simulink model "motivation"  (R2021b)
settings: Solver=FixedStepAuto  StartTime=0.0  StopTime=simTime  FixedStep=simStep  RelTol=1e-3
values from neighbouring files (symbols this model uses):
  Delta = 0.1    [init.m]
  Gain = place(A,b, [-3 , -10])    [init.m]
  Gains = place(As, bs, [0.2 , 0.1])    [init.m]
  k1 = 1    [init.m]
  k2 = 1    [init.m]
  simStep = 10^-4    (= 0.0001)    [init.m]
  x0 = [-1;1]    [init.m]
settings Model: Creator=mebbaid  LastModifiedBy=mebbaid

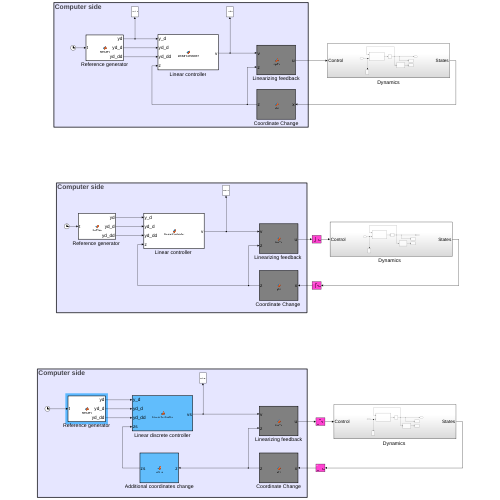
[thumbnail: Simulink's stored preview of the top-level diagram]
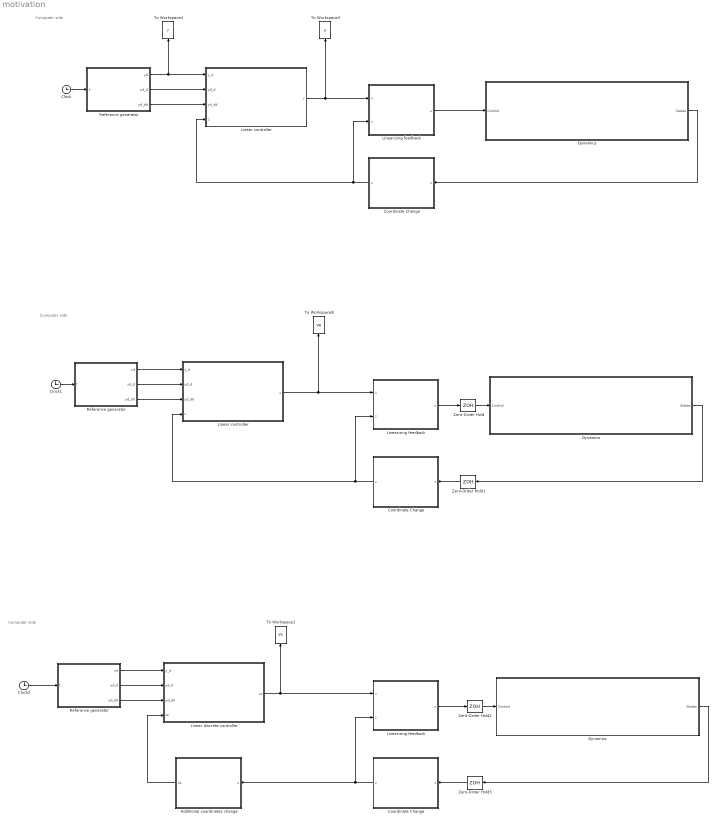
== system motivation ==
  note: Computer side
  note: Computer side
  note: Computer side
  " Coordinate Change " : MATLAB Function  TreatAsAtomicUnit=on
  " Dynamics  " : Subsystem
  " Linearizing feedback " : MATLAB Function  TreatAsAtomicUnit=on
  " Reference generator " : MATLAB Function  TreatAsAtomicUnit=on
  Additional coordinates change : MATLAB Function  TreatAsAtomicUnit=on
  Clock : Clock
  Clock1 : Clock
  Clock2 : Clock
  Coordinate Change : MATLAB Function  TreatAsAtomicUnit=on
  "Coordinate Change " : MATLAB Function  TreatAsAtomicUnit=on
  Dynamics : Subsystem
  "Dynamics  " : Subsystem
  Linear controller : MATLAB Function  TreatAsAtomicUnit=on
  "Linear controller " : MATLAB Function  TreatAsAtomicUnit=on
  Linear discrete controller : MATLAB Function  TreatAsAtomicUnit=on
  Linearizing feedback : MATLAB Function  TreatAsAtomicUnit=on
  "Linearizing feedback " : MATLAB Function  TreatAsAtomicUnit=on
  Reference generator : MATLAB Function  TreatAsAtomicUnit=on
  "Reference generator " : MATLAB Function  TreatAsAtomicUnit=on
  To Workspace1 : ToWorkspace  VariableName=vs  SaveFormat=Timeseries  SampleTime=simStep
      settings: Save2DSignal=2-D array (concatenate along first dimension)
  To Workspace3 : ToWorkspace  VariableName=v  SaveFormat=Timeseries  SampleTime=simStep
      settings: Save2DSignal=2-D array (concatenate along first dimension)
  To Workspace4 : ToWorkspace  VariableName=r  SaveFormat=Timeseries  SampleTime=simStep
      settings: Save2DSignal=2-D array (concatenate along first dimension)
  To Workspace8 : ToWorkspace  VariableName=ve  SaveFormat=Timeseries  SampleTime=simStep
      settings: Save2DSignal=2-D array (concatenate along first dimension)
  Zero-Order Hold{,1..3} (4 alike) : ZeroOrderHold  SampleTime=Delta
  wires:
  Linear controller/1(v) -> Linearizing feedback/1(v), To Workspace3/1
  Clock/1 -> Reference generator/1(t)
  Reference generator/3(yd_dd) -> Linear controller/3(yd_dd)
  Reference generator/1(yd) -> Linear controller/1(y_d), To Workspace4/1
  Reference generator/2(yd_d) -> Linear controller/2(yd_d)
  Linearizing feedback/1(u) -> Dynamics/1(Control)
  Coordinate Change/1(z) -> Linear controller/4(z), Linearizing feedback/2(z)
  Dynamics/1(States) -> Coordinate Change/1(x)
  "Linearizing feedback "/1(u) -> Zero-Order Hold/1
  "Dynamics  "/1(States) -> Zero-Order Hold1/1
  "Linear controller "/1(v) -> "Linearizing feedback "/1(v), To Workspace8/1
  "Coordinate Change "/1(z) -> "Linear controller "/4(z), "Linearizing feedback "/2(z)
  "Reference generator "/1(yd) -> "Linear controller "/1(y_d)
  "Reference generator "/2(yd_d) -> "Linear controller "/2(yd_d)
  "Reference generator "/3(yd_dd) -> "Linear controller "/3(yd_dd)
  Clock1/1 -> "Reference generator "/1(t)
  Zero-Order Hold/1 -> "Dynamics  "/1(Control)
  Zero-Order Hold1/1 -> "Coordinate Change "/1(x)
  Zero-Order Hold2/1 -> " Dynamics  "/1(Control)
  " Dynamics  "/1(States) -> Zero-Order Hold3/1
  " Linearizing feedback "/1(u) -> Zero-Order Hold2/1
  Zero-Order Hold3/1 -> " Coordinate Change "/1(x)
  " Coordinate Change "/1(z) -> " Linearizing feedback "/2(z), Additional coordinates change/1(z)
  Linear discrete controller/1(vs) -> " Linearizing feedback "/1(v), To Workspace1/1
  " Reference generator "/3(yd_dd) -> Linear discrete controller/3(yd_dd)
  " Reference generator "/2(yd_d) -> Linear discrete controller/2(yd_d)
  " Reference generator "/1(yd) -> Linear discrete controller/1(y_d)
  Clock2/1 -> " Reference generator "/1(t)
  Additional coordinates change/1(zs) -> Linear discrete controller/4(zs)

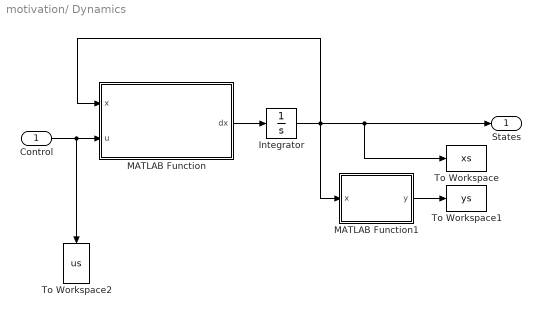
== system motivation/ Dynamics   ==
  Control : Inport
  Integrator : Integrator  InitialCondition=x0
  MATLAB Function : MATLAB Function  TreatAsAtomicUnit=on
  MATLAB Function1 : MATLAB Function  TreatAsAtomicUnit=on
  To Workspace : ToWorkspace  VariableName=xs  SaveFormat=Timeseries  SampleTime=simStep
      settings: Save2DSignal=2-D array (concatenate along first dimension)
  To Workspace1 : ToWorkspace  VariableName=ys  SaveFormat=Timeseries  SampleTime=simStep
      settings: Save2DSignal=2-D array (concatenate along first dimension)
  To Workspace2 : ToWorkspace  VariableName=us  SaveFormat=Timeseries  SampleTime=simStep
      settings: Save2DSignal=2-D array (concatenate along first dimension)
  States : Outport
  wires:
  MATLAB Function/1(dx) -> Integrator/1
  MATLAB Function1/1(y) -> To Workspace1/1
  Control/1 -> MATLAB Function/2(u), To Workspace2/1
  Integrator/1 -> To Workspace/1, States/1, MATLAB Function/1(x), MATLAB Function1/1(x)

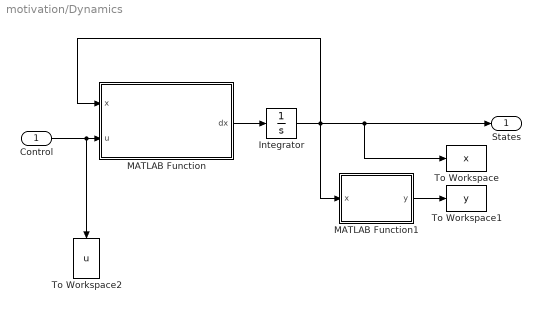
== system motivation/Dynamics ==
  Control : Inport
  Integrator : Integrator  InitialCondition=x0
  MATLAB Function : MATLAB Function  TreatAsAtomicUnit=on
  MATLAB Function1 : MATLAB Function  TreatAsAtomicUnit=on
  To Workspace : ToWorkspace  VariableName=x  SaveFormat=Timeseries  SampleTime=simStep
      settings: Save2DSignal=2-D array (concatenate along first dimension)
  To Workspace1 : ToWorkspace  VariableName=y  SaveFormat=Timeseries  SampleTime=simStep
      settings: Save2DSignal=2-D array (concatenate along first dimension)
  To Workspace2 : ToWorkspace  VariableName=u  SaveFormat=Timeseries  SampleTime=simStep
      settings: Save2DSignal=2-D array (concatenate along first dimension)
  States : Outport
  wires:
  MATLAB Function/1(dx) -> Integrator/1
  MATLAB Function1/1(y) -> To Workspace1/1
  Control/1 -> To Workspace2/1, MATLAB Function/2(u)
  Integrator/1 -> To Workspace/1, States/1, MATLAB Function/1(x), MATLAB Function1/1(x)

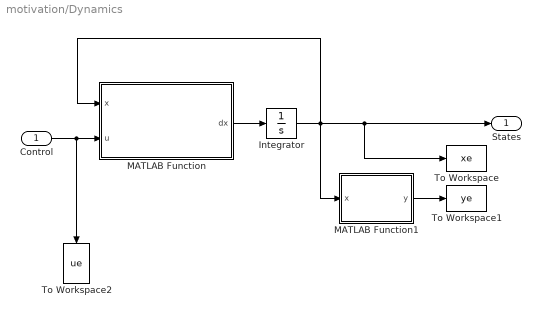
== system motivation/Dynamics   ==
  Control : Inport
  Integrator : Integrator  InitialCondition=x0
  MATLAB Function : MATLAB Function  TreatAsAtomicUnit=on
  MATLAB Function1 : MATLAB Function  TreatAsAtomicUnit=on
  To Workspace : ToWorkspace  VariableName=xe  SaveFormat=Timeseries  SampleTime=simStep
      settings: Save2DSignal=2-D array (concatenate along first dimension)
  To Workspace1 : ToWorkspace  VariableName=ye  SaveFormat=Timeseries  SampleTime=simStep
      settings: Save2DSignal=2-D array (concatenate along first dimension)
  To Workspace2 : ToWorkspace  VariableName=ue  SaveFormat=Timeseries  SampleTime=simStep
      settings: Save2DSignal=2-D array (concatenate along first dimension)
  States : Outport
  wires:
  MATLAB Function/1(dx) -> Integrator/1
  MATLAB Function1/1(y) -> To Workspace1/1
  Control/1 -> MATLAB Function/2(u), To Workspace2/1
  Integrator/1 -> To Workspace/1, States/1, MATLAB Function/1(x), MATLAB Function1/1(x)

== matlab function motivation/Coordinate Change  ==
  data: x input; z output
function z = phi(x)
x_1 = x(1);
x_2 = x(2);
z = [2*x_1 + cos(x_1);
     x_2 - sin(x_1)];

== matlab function motivation/Reference generator  ==
  data: t input; yd output; yd_d output; yd_dd output; refType parameter
function [yd, yd_d, yd_dd] = RefGen(t, refType)

if refType==1
    yd   = sin(t);
    yd_d = cos(t);
    yd_dd = -sin(t);
else
    yd = 3.5;
    yd_d = 0;
    yd_dd =  0;
end

== matlab function motivation/ Dynamics  /MATLAB Function ==
  data: x input; u input; dx output
function dx = dynamics(x, u)
x_1 = x(1);
x_2 = x(2);

dx = [-1/(sin(x_1)-2)*(x_2 - sin(x_1));
      -2*x_1 - x_2 - (cos(x_1)*(x_2-sin(x_1)))/(sin(x_1)-2) - ...
      cos(x_1) + sin(x_1) + (2*x_1 + cos(x_1))*(x_2 - sin(x_1)) + u];

== matlab function motivation/ Dynamics  /MATLAB Function1 ==
  data: x input; y output
function y = outputFunc(x)

y =  2*x(1) + cos(x(1));

== matlab function motivation/ Linearizing feedback  ==
  data: v input; z input; u output
function u = inpTx(v, z)
z_1 = z(1);
z_2 = z(2);

u = -z_1*z_2 + v;

== matlab function motivation/ Coordinate Change  ==
  data: x input; z output
function z = phi(x)
x_1 = x(1);
x_2 = x(2);
z = [2*x_1 + cos(x_1);
     x_2 - sin(x_1)];

== matlab function motivation/Dynamics/MATLAB Function1 ==
  data: x input; y output
function y = outputFunc(x)

y = 2*x(1) + cos(x(1));

== matlab function motivation/Additional coordinates change ==
  data: z input; zs output; Delta parameter
function zs = phi_s(z, Delta)
Ts = [1 -Delta/2;0 1];
zs = Ts * z;

== matlab function motivation/Linear discrete controller ==
  data: y_d input; yd_d input; yd_dd input; zs input; vs output; k1 parameter; k2 parameter; Gains parameter
function vs = LinearController( y_d, yd_d,yd_dd, zs, k1, k2, Gains)
z_1 = zs(1);
z_2 = zs(2);

% -------- normal linear control design using error system
e    = [z_1 - y_d; z_2 - yd_d]; 
vs   = -Gains*e;
% v =   yd_dd + k2*(yd_d - z_2) + k1*(y_d - z_1);

== matlab function motivation/ Reference generator  ==
  data: t input; yd output; yd_d output; yd_dd output; refType parameter
function [yd, yd_d, yd_dd] = RefGen(t, refType)

if refType==1
    yd   = sin(t);
    yd_d = cos(t);
    yd_dd = -sin(t);
else
    yd = 3.5;
    yd_d = 0;
    yd_dd =  0;
end

== matlab function motivation/Dynamics/MATLAB Function ==
  data: x input; u input; dx output
function dx = dynamics(x, u)
x_1 = x(1);
x_2 = x(2);

dx = [-1/(sin(x_1)-2)*(x_2 - sin(x_1));
      -2*x_1 - x_2 - (cos(x_1)*(x_2-sin(x_1)))/(sin(x_1)-2) - ...
      cos(x_1) + sin(x_1) + (2*x_1 + cos(x_1))*(x_2 - sin(x_1)) + u];

== matlab function motivation/Coordinate Change ==
  data: x input; z output
function z = phi(x)
x_1 = x(1);
x_2 = x(2);
z = [2*x_1 + cos(x_1);
     x_2 - sin(x_1)];

== matlab function motivation/Linearizing feedback ==
  data: v input; z input; u output
function u = inpTx(v, z)
z_1 = z(1);
z_2 = z(2);

u = -z_1*z_2 + v;

== matlab function motivation/Linear controller ==
  data: y_d input; yd_d input; yd_dd input; z input; v output; k1 parameter; k2 parameter; Gain parameter
function v = LinearController( y_d, yd_d,yd_dd, z, k1, k2, Gain)
z_1 = z(1);
z_2 = z(2);

% -------- normal linear control design using error system
e    = [z_1 - y_d; z_2 - yd_d]; 
v    = -Gain*e;
% v =   yd_dd + k2*(yd_d - z_2) + k1*(y_d - z_1);

== matlab function motivation/Reference generator ==
  data: t input; yd output; yd_d output; yd_dd output; refType parameter
function [yd, yd_d, yd_dd] = RefGen(t, refType)

if refType==1
    yd   = sin(t);
    yd_d = cos(t);
    yd_dd = -sin(t);
else
    yd = 3.5;
    yd_d = 0;
    yd_dd =  0;
end

== matlab function motivation/Linear controller  ==
  data: y_d input; yd_d input; yd_dd input; z input; v output; k1 parameter; k2 parameter; Gain parameter
function v = LinearController( y_d, yd_d,yd_dd, z, k1, k2, Gain)
z_1 = z(1);
z_2 = z(2);

% -------- normal linear control design using error system
e    = [z_1 - y_d; z_2 - yd_d]; 
v    = -Gain*e;
% v =   yd_dd + k2*(yd_d - z_2) + k1*(y_d - z_1);

== matlab function motivation/Dynamics  /MATLAB Function ==
  data: x input; u input; dx output
function dx = dynamics(x, u)
x_1 = x(1);
x_2 = x(2);

dx = [-1/(sin(x_1)-2)*(x_2 - sin(x_1));
      -2*x_1 - x_2 - (cos(x_1)*(x_2-sin(x_1)))/(sin(x_1)-2) - ...
      cos(x_1) + sin(x_1) + (2*x_1 + cos(x_1))*(x_2 - sin(x_1)) + u];

== matlab function motivation/Dynamics  /MATLAB Function1 ==
  data: x input; y output
function y = outputFunc(x)

y =  2*x(1) + cos(x(1));

== matlab function motivation/Linearizing feedback  ==
  data: v input; z input; u output
function u = inpTx(v, z)
z_1 = z(1);
z_2 = z(2);

u = -z_1*z_2 + v;
